simulink model "DTNS_SIM2"  (R2022a)
settings: Solver=ode4  StartTime=0.0  StopTime=100  FixedStep=0.01  RelTol=1e-3  EnableMultiTasking=on
PreLoadFcn:
  | listing = dir;
  | if (contains([listing.name], 'MAP')) &&  (contains([listing.name], 'DTNS_SIM.slx'))
  |     addpath('./AGR', './TRN', './TCAF', './FTG', './DYN', './FLCC', './GPS', './RALT', './INS', './MAP');
  |     addpath('./MAP/MAP_DB');
  | else
  |     warning('[DTNS_SIM.slx]는 DTNS 프로젝트 최상단 경로에 위치해야 합니다.');
  | end
  | 
  | load('BUS_STRUCTURE_DYN.mat');
  | load('BUS_STRUCTURE_FLCC.mat');
  | load('BUS_STRUCTURE_RALT.mat');
  | load('BUS_STRUCTURE_INS.mat');
  | load('BUS_STRUCTURE_GPS.mat');
  | load('BusStructureTRN.mat');
  | load('BusStructureLOSR.mat');
  | load('BusStructureHR.mat');
  | load('BusStructureCR.mat');
  | FTG_initState;
InitFcn:
  | listing = dir;
  | if (contains([listing.name], 'MAP')) &&  (contains([listing.name], 'DTNS_SIM.slx'))
  |     addpath('./AGR', './TRN', './TCAF', './FTG', './DYN', './FLCC', './GPS', './RALT', './INS', './MAP');
  |     addpath('./MAP/MAP_DB');
  | else
  |     warning('[DTNS_SIM.slx]는 DTNS 프로젝트 최상단 경로에 위치해야 합니다.');
  | end
  | 
  | load('BUS_STRUCTURE_DYN.mat');
  | load('BUS_STRUCTURE_FLCC.mat');
  | load('BUS_STRUCTURE_RALT.mat');
  | load('BUS_STRUCTURE_INS.mat');
  | load('BUS_STRUCTURE_GPS.mat');
  | load('BusStructureTRN.mat');
  | load('BusStructureLOSR.mat');
  | load('BusStructureHR.mat');
  | load('BusStructureCR.mat');
  | FTG_initState;
libraries: aerolibconvert2 x14, simulink_extras x5
(part 1 of 2)
settings Model: PacingRate=3  Creator=ASCL  LastModifiedBy=ASCL
settings SolverCC: PositivePriorityOrder=on  AutoInsertRateTranBlk=on
settings DataIOCC: ExternalInput=FTGScenario.getElement('IN_STICK'), [], [], FTGScenario.getElement('IN_FLIGHT_CMD'), []  LoadExternalInput=on  SaveOutput=off  DSMLogging=off  ReturnWorkspaceOutputs=off
settings OptimizationCC: BlockReduction=off  DefaultParameterBehavior=Inlined  UseDivisionForNetSlopeComputation=on  GainParamInheritBuiltInType=on  UseFloatMulNetSlope=on  ExpressionFolding=off  PassReuseOutputArgsAs=Individual arguments  ZeroExternalMemoryAtStartup=off  ZeroInternalMemoryAtStartup=off  EfficientFloat2IntCast=on  LifeSpan=inf  OptimizeBlockOrder=speed  DifferentSizesBufferReuse=on  EfficientTunableParamExpr=on
settings DebuggingCC: SignalInfNanChecking=warning  ReadBeforeWriteMsg=EnableAllAsError  WriteAfterWriteMsg=EnableAllAsError  WriteAfterReadMsg=EnableAllAsError  IntegerOverflowMsg=error  ParameterTunabilityLossMsg=error  UniqueDataStoreMsg=error  AssertControl=DisableAll  NonBusSignalsTreatedAsBus=error  SFInvalidInputDataAccessInChartInitDiag=error  SFTransitionOutsideNaturalParentDiag=error  SFUnreachableExecutionPathDiag=error  SFUndirectedBroadcastEventsDiag=error  IntegerSaturationMsg=error
settings HardwareCC: ProdBitPerPointer=32  ProdBitPerSizeT=32  ProdBitPerPtrDiffT=32  ProdLargestAtomicInteger=Long  ProdLargestAtomicFloat=Double  ProdEndianess=BigEndian  ProdWordSize=32  ProdLongLongMode=on  ProdHWDeviceType=Freescale->MPC83xx
settings ModelReferenceCC: ModelReferenceNumInstancesAllowed=Single
settings SFSimCC: SimCustomHeaderCode="#include \"MAP.h\""  SimUserSources=MAP.c  SimUserLibraries=WS2_32.LIB  CompileTimeRecursionLimit=0  EnableRuntimeRecursion=off  MATLABDynamicMemAlloc=off  CustomCodeGlobalsAsFunctionIO=on
settings RTWCC: SystemTargetFile=ert.tlc  TemplateMakefile=ert_default_tmf  GenerateReport=on  RTWUseSimCustomCode=on  CustomHeaderCode="#include \"MAP.h\""  CustomSource=MAP.c  CustomLibrary=WS2_32.LIB  BuildConfiguration=Faster Runs  IncludeHyperlinkInReport=on  LaunchReport=on  GenerateTraceInfo=on  GenerateTraceReport=on  GenerateTraceReportSl=on  GenerateTraceReportSf=on  GenerateTraceReportEml=on  GenerateCodeMetricsReport=on
settings CodeAppCC: ForceParamTrailComments=on  IgnoreCustomStorageClasses=off  OperatorAnnotations=on  SimulinkDataObjDesc=on  SFDataObjDesc=on  MATLABFcnDesc=on  InsertBlockDesc=on  StateflowObjectComments=on  MATLABSourceComments=on  EnableCustomComments=on  InlinedPrmAccess=Macros  ReqsInCode=on
settings ERTTargetCC: TargetLangStandard=C99 (ISO)  UtilityFuncGeneration=Shared location  GenerateSampleERTMain=on  CombineSignalStateStructs=on  SuppressErrorStatus=on  SupportNonFinite=off  SupportVariableSizeSignals=on  ParenthesesLevel=Standards  CastingMode=Standards  GenerateSharedConstants=off  InlinedParameterPlacement=NonHierarchical  ERTCustomFileTemplate=example_file_process.tlc  RateTransitionBlockCode=Function  PreserveIfCondition=on  ConvertIfToSwitch=off  EnableSignedLeftShifts=off  EnableSignedRightShifts=off

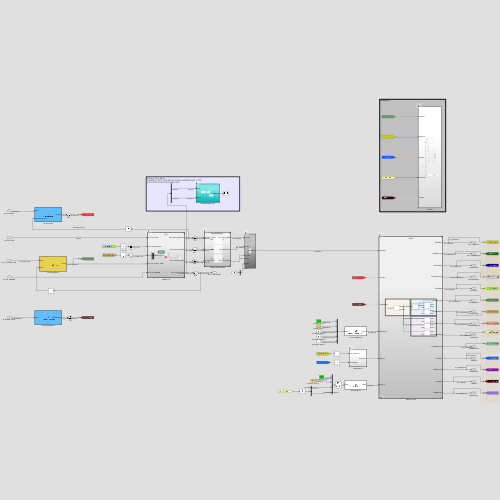
[thumbnail: Simulink's stored preview of the top-level diagram]
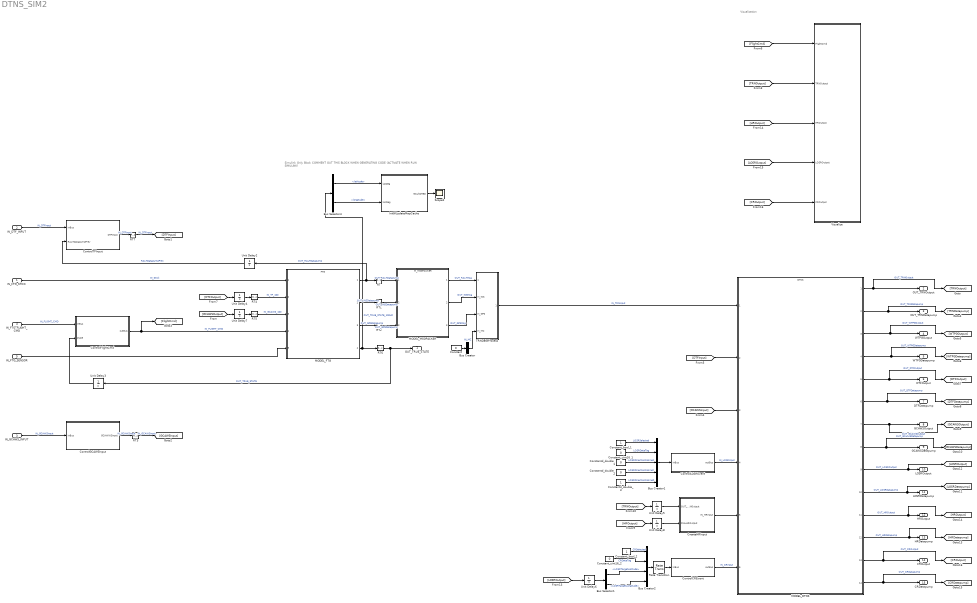
== system DTNS_SIM2 ==
  note: Visualization
  note: Simulink Only Block
      | COMMENT OUT THIS BLOCK WHEN GENERATING CODE
      | (ACTIVATE WHEN RUN SIMULINK)
  IN_FTG_STICK : Inport  OutDataTypeStr=Bus: BUS_FLCC_STICK  BusOutputAsStruct=on
  IN_DTF_INPUT : Inport  Port=2  OutDataTypeStr=Bus: DTFInput  BusOutputAsStruct=on
  IN_GCAWS_INPUT : Inport  Port=3  OutDataTypeStr=Bus: GCAWSInput  BusOutputAsStruct=on
  IN_FTG_FLIGHT_CMD : Inport  Port=4  OutDataTypeStr=Bus: BUS_FLCC_FLIGHT_CMD  Interpolate=off  BusOutputAsStruct=on
  IN_FTG_SENSOR : Inport  Port=5  OutDataTypeStr=Bus: BUS_SENSOR_ALL_INPUTSTATUS  BusOutputAsStruct=on
  Bus Creator : BusCreator  Inputs=1  OutDataTypeStr=Bus: TRN_MC  NonVirtualBus=on
      settings: InheritFromInputs=off
  Bus Creator1 : BusCreator  Inputs=5  OutDataTypeStr=Bus: LOSRInput  NonVirtualBus=on
      settings: InheritFromInputs=off
  Bus Creator2 : BusCreator  Inputs=4  OutDataTypeStr=Bus: CRInput
      settings: InheritFromInputs=off
  Bus Selector1 : BusSelector  OutputSignals=LOSRTargetLatitude,LOSRTargetLongitude
  Bus Selector4 : BusSelector  OutputSignals=latitude,longitude
  Constant : Constant  Value=0  OutDataTypeStr=boolean  SampleTime=0.04
  Constant_bool_1 : Constant  OutDataTypeStr=boolean  SampleTime=0.04
  Constant_bool_2 : Constant  OutDataTypeStr=boolean  SampleTime=0.04
  Constant_uint16_1 : Constant  Value=0  OutDataTypeStr=uint16  SampleTime=0.04
  Constant_uint16_2 : Constant  Value=0  OutDataTypeStr=uint16  SampleTime=0.04
  Constantd_double_1 : Constant  Value=0  OutDataTypeStr=double  SampleTime=0.04
  Constantd_double_2 : Constant  Value=0  OutDataTypeStr=double  SampleTime=0.04
  Constantd_double_3 : Constant  OutDataTypeStr=double  SampleTime=0.04
  ControlCREvent : MATLAB Function  TreatAsAtomicUnit=on  SystemSampleTime=0.04
  ControlFlightCmd : MATLAB Function  TreatAsAtomicUnit=on  SystemSampleTime=0.01
  ControlGCAWSInput : MATLAB Function  TreatAsAtomicUnit=on  SystemSampleTime=0.01
  ControlLOSREvent : MATLAB Function  TreatAsAtomicUnit=on  SystemSampleTime=0.04
  ControlTFInput : MATLAB Function  TreatAsAtomicUnit=on  SystemSampleTime=0.01
  CreateHRInput : Subsystem  TreatAsAtomicUnit=on  ScheduleAs=Periodic partition  PartitionName=CreateHRInput  SystemSampleTime=0.04
      settings: RTWSystemCode=Nonreusable function
  InitNUpdateMapCache : Subsystem  TreatAsAtomicUnit=on  ScheduleAs=Periodic partition  PartitionName=InitNUpdateMapCache  SystemSampleTime=0.01
  MODEL_DTNS : ModelReference  ModelNameDialog=DTNS.slx  SimulationMode=Normal  ScheduleRates=on  ScheduleRatesWith=Schedule Editor  ModelReferenceVersion=1.240
  MODEL_FTG : ModelReference  ModelNameDialog=FTG.slx  SimulationMode=Normal  ScheduleRates=on  ScheduleRatesWith=Schedule Editor  ModelReferenceVersion=1.515
  MODEL_MSGPACKER : ModelReference  ModelNameDialog=M_MSGPACKER.slx  SimulationMode=Normal  ScheduleRates=on  ScheduleRatesWith=Schedule Editor  ModelReferenceVersion=1.319
  RT{,1..3,6..7} (6 alike) : RateTransition  OutPortSampleTime=0.04
  RT4 : RateTransition  OutPortSampleTime=0.01
  RT5 : RateTransition  OutPortSampleTime=0.01
  Rate Transition : RateTransition  OutPortSampleTime=0.04
  Scope2 : Scope
  TRNDataProcess : Subsystem  TreatAsAtomicUnit=on  ScheduleAs=Periodic partition  PartitionName=TRNDataProcess  SystemSampleTime=0.04
  Unit Delay2 : UnitDelay  SampleTime=0.01  HasFrameUpgradeWarning=on
  Unit Delay3 : UnitDelay  SampleTime=-1  HasFrameUpgradeWarning=on
  Unit Delay{4..8} (5 alike) : UnitDelay  SampleTime=0.04  HasFrameUpgradeWarning=on
  Visualize : Subsystem  TreatAsAtomicUnit=on  ScheduleAs=Periodic partition  PartitionName=Visualize  SystemSampleTime=0.04
  OUT_TRUE_STATE : Outport  OutDataTypeStr=Bus: BUS_DYN_STATE  BusOutputAsStruct=on
  OUT_TRNOutput : Outport  Port=2  OutDataTypeStr=Bus: TRNOutput  SampleTime=0.04
  OUT_TRNDatapump : Outport  Port=3  OutDataTypeStr=Bus: TRNDatapump  SampleTime=0.04
  WTPGOutput : Outport  Port=4  OutDataTypeStr=Bus: WTPGOutput  SampleTime=0.04
  WTPGDatapump : Outport  Port=5  OutDataTypeStr=Bus: WTPGDatapump  SampleTime=0.04
  DTFOutput : Outport  Port=6  OutDataTypeStr=Bus: DTFOutput  SampleTime=0.04
  DTFDatapump : Outport  Port=7  OutDataTypeStr=Bus: DTFDatapump  SampleTime=0.04
  GCAWSOutput : Outport  Port=8  OutDataTypeStr=Bus: GCAWSOutput  SampleTime=0.04
  GCAWSDatapump : Outport  Port=9  OutDataTypeStr=Bus: GCAWSDatapump  SampleTime=0.04
  LOSROutput : Outport  Port=10  OutDataTypeStr=Bus: LOSROutput  SampleTime=0.04  BusOutputAsStruct=on
  LOSRDatapump : Outport  Port=11  OutDataTypeStr=Bus: LOSRDatapump  SampleTime=0.04  BusOutputAsStruct=on
  HROutput : Outport  Port=12  OutDataTypeStr=Bus: HROutput  SampleTime=0.04  BusOutputAsStruct=on
  HRDatapump : Outport  Port=13  OutDataTypeStr=Bus: HRDatapump  SampleTime=0.04  BusOutputAsStruct=on
  CROutput : Outport  Port=14  OutDataTypeStr=Bus: CROutput  SampleTime=0.04  BusOutputAsStruct=on
  CRDatapump : Outport  Port=15  OutDataTypeStr=Bus: CRDatapump  SampleTime=0.04  BusOutputAsStruct=on
  wires:
  Bus Creator/1 -> TRNDataProcess/4(In_MC)  "IN_MC"
  MODEL_FTG/3 -> RT2/1  "OUT_GPSDatapump"
  MODEL_DTNS/4 -> [WTPGDatapump], WTPGDatapump/1  "OUT_WTPGDatapump"
  MODEL_DTNS/8 -> [GCAWSDatapump], GCAWSDatapump/1  "OUT_GCAWSDatapump"
  MODEL_DTNS/2 -> [TRNDatapump], OUT_TRNDatapump/1  "OUT_TRNDatapump"
  MODEL_DTNS/7 -> GCAWSOutput/1, [GCAWSOutput]  "OUT_GCAWSOutput"
  Constant/1 -> Bus Creator/1
  IN_GCAWS_INPUT/1 -> ControlGCAWSInput/1(inBus)  "IN_GCAWSInput"
  IN_FTG_FLIGHT_CMD/1 -> ControlFlightCmd/1(inBus)  "IN_FLIGHT_CMD"
  RT6/1 -> Unit Delay3/1, OUT_TRUE_STATE/1  "OUT_TRUE_STATE"
  Bus Selector4/2 -> InitNUpdateMapCache/2(lonDeg)  "<longitude>"
  MODEL_FTG/2 -> RT1/1  "OUT_INSDatapump"
  MODEL_FTG/1 -> RT/1, Unit Delay2/1  "OUT_RALTDatapump"
  IN_FTG_STICK/1 -> MODEL_FTG/1  "IN_Stick"
  MODEL_DTNS/5 -> DTFOutput/1, [DTFOutput]  "OUT_DTFOutput"
  ControlFlightCmd/1(outBus) -> MODEL_FTG/4, [FlightCmd]  "IN_FLIGHT_CMD"
  IN_DTF_INPUT/1 -> ControlTFInput/1(inBus)  "IN_DTFInput"
  MODEL_MSGPACKER/3 -> TRNDataProcess/3(In_GPS)  "OUT_GPSMsg"
  MODEL_MSGPACKER/1 -> TRNDataProcess/1(In_RALT)  "OUT_RALTMsg"
  MODEL_MSGPACKER/2 -> TRNDataProcess/2(In_INS)  "OUT_INSMsg"
  InitNUpdateMapCache/1(resultDTED) -> Scope2/1
  IN_FTG_SENSOR/1 -> MODEL_FTG/5
  RT7/1 -> [DTFInput]  "IN_DTFInput"
  Unit Delay2/1 -> ControlTFInput/2(RALTDatapumpPrev)  "RALTDatapumpPrev"
  RT3/1 -> [GCAWSInput]  "IN_GCAWSInput"
  Unit Delay3/1 -> ControlFlightCmd/2(state)
  TRNDataProcess/1(TRN INPUT) -> MODEL_DTNS/1  "IN_TRNInput"
  RT/1 -> MODEL_MSGPACKER/1  "OUT_RALTDatapump"
  RT1/1 -> MODEL_MSGPACKER/2  "OUT_INSDatapump"
  RT2/1 -> MODEL_MSGPACKER/3  "OUT_GPSDatapump"
  Bus Selector4/1 -> InitNUpdateMapCache/1(latDeg)  "<latitude>"
  RT4/1 -> MODEL_FTG/2  "IN_TF_100"
  RT5/1 -> MODEL_FTG/3  "IN_GCAWS_100"
  MODEL_FTG/4 -> Bus Selector4/1, RT6/1  "OUT_TRUE_STATE_100HZ"
  MODEL_DTNS/12 -> [HRDatapump], HRDatapump/1  "OUT_HRDatapump"
  Bus Creator1/1 -> ControlLOSREvent/1(inBus)
  Constant_uint16_1/1 -> Bus Creator1/2  "LOSRDataTag"
  MODEL_DTNS/9 -> LOSROutput/1, [LOSROutput]  "OUT_LOSROutput"
  MODEL_DTNS/1 -> [TRNOutput], OUT_TRNOutput/1  "OUT_TRNOutput"
  MODEL_DTNS/14 -> [CRDatapump], CRDatapump/1  "OUT_CRDatapump"
  MODEL_DTNS/13 -> [CROutput], CROutput/1  "OUT_CROutput"
  Constantd_double_2/1 -> Bus Creator1/4  "LOSRDirectionCosineY"
  Constant_bool_1/1 -> Bus Creator1/1  "LOSRSelected"
  ControlLOSREvent/1(outBus) -> MODEL_DTNS/4  "IN_LOSRInput"
  Constantd_double_3/1 -> Bus Creator1/5  "LOSRDirectionCosineZ"
  Constantd_double_1/1 -> Bus Creator1/3  "LOSRDirectionCosineX"
  MODEL_DTNS/10 -> [LOSRDatapump], LOSRDatapump/1  "OUT_LOSRDatapump"
  MODEL_DTNS/6 -> [DTFDatapump], DTFDatapump/1  "OUT_DTFDatapump"
  CreateHRInput/1(IN_HRInput) -> MODEL_DTNS/5
  MODEL_DTNS/3 -> [WTPGOutput], WTPGOutput/1  "OUT_WTPGOutput"
  MODEL_DTNS/11 -> [HROutput], HROutput/1  "OUT_HROutput"
  [TRNOutput] -> Visualize/2(TRNOutput)
  [FlightCmd] -> Visualize/1(FlightCmd)
  [HROutput] -> Visualize/3(HROutput)
  [LOSROutput] -> Visualize/4(LOSROutput)
  [CROutput] -> Visualize/5(CROutput)
  [TRNOutput] -> Unit Delay5/1
  ControlGCAWSInput/1(GCAWWSInput) -> RT3/1  "IN_GCAWSInput"
  ControlTFInput/1(DTFInput) -> RT7/1  "IN_DTFInput"
  [DTFInput] -> MODEL_DTNS/2
  [GCAWSInput] -> MODEL_DTNS/3
  Unit Delay5/1 -> CreateHRInput/1(OUT_TRNOutput)
  Bus Selector1/2 -> Bus Creator2/4  "<LOSRTargetLongitude>"
  [LOSROutput] -> Unit Delay6/1
  Rate Transition/1 -> ControlCREvent/1(inBus)
  Bus Selector1/1 -> Bus Creator2/3  "<LOSRTargetLatitude>"
  Bus Creator2/1 -> Rate Transition/1
  ControlCREvent/1(outBus) -> MODEL_DTNS/6  "IN_CRInput"
  Constant_bool_2/1 -> Bus Creator2/1  "CRSelected"
  Constant_uint16_2/1 -> Bus Creator2/2  "CRDataTag"
  Unit Delay6/1 -> Bus Selector1/1
  [DTFOutput] -> Unit Delay4/1
  Unit Delay4/1 -> RT4/1
  Unit Delay7/1 -> RT5/1
  [HROutput] -> Unit Delay8/1
  Unit Delay8/1 -> CreateHRInput/2(PrevHROutput)
  [GCAWSOutput] -> Unit Delay7/1

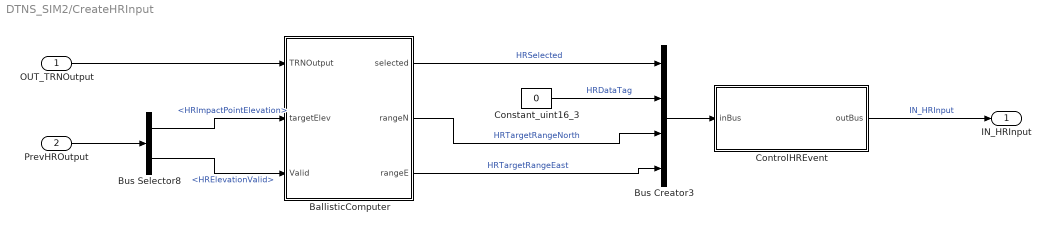
== system DTNS_SIM2/CreateHRInput ==
  OUT_TRNOutput : Inport
  PrevHROutput : Inport  Port=2
  BallisticComputer : MATLAB Function  TreatAsAtomicUnit=on  SystemSampleTime=0.04
  Bus Creator3 : BusCreator  Inputs=4  OutDataTypeStr=Bus: HRInput  NonVirtualBus=on
      settings: InheritFromInputs=off
  Bus Selector8 : BusSelector  OutputSignals=HRImpactPointElevation,HRElevationValid
  Constant_uint16_3 : Constant  Value=0  OutDataTypeStr=uint16  SampleTime=0.04
  ControlHREvent : MATLAB Function  TreatAsAtomicUnit=on  SystemSampleTime=0.04
  IN_HRInput : Outport
  wires:
  BallisticComputer/3(rangeE) -> Bus Creator3/4  "HRTargetRangeEast"
  BallisticComputer/2(rangeN) -> Bus Creator3/3  "HRTargetRangeNorth"
  Bus Selector8/1 -> BallisticComputer/2(targetElev)  "<HRImpactPointElevation>"
  BallisticComputer/1(selected) -> Bus Creator3/1  "HRSelected"
  OUT_TRNOutput/1 -> BallisticComputer/1(TRNOutput)
  Constant_uint16_3/1 -> Bus Creator3/2  "HRDataTag"
  Bus Creator3/1 -> ControlHREvent/1(inBus)
  Bus Selector8/2 -> BallisticComputer/3(Valid)  "<HRElevationValid>"
  PrevHROutput/1 -> Bus Selector8/1
  ControlHREvent/1(outBus) -> IN_HRInput/1  "IN_HRInput"

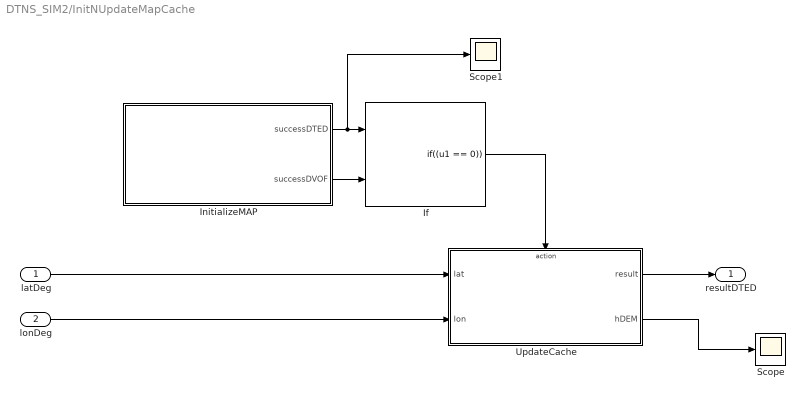
== system DTNS_SIM2/InitNUpdateMapCache ==
  latDeg : Inport  OutDataTypeStr=double
  lonDeg : Inport  Port=2  OutDataTypeStr=double
  If : If  NumInputs=2  IfExpression=(u1 == 0)  ShowElse=off
  InitializeMAP : MATLAB Function  TreatAsAtomicUnit=on
  Scope : Scope
  Scope1 : Scope
  UpdateCache : Subsystem  TreatAsAtomicUnit=on
  resultDTED : Outport  VectorParamsAs1DForOutWhenUnconnected=off
  wires:
  lonDeg/1 -> UpdateCache/2(lon)
  UpdateCache/1(result) -> resultDTED/1
  InitializeMAP/1(successDTED) -> Scope1/1, If/1
  latDeg/1 -> UpdateCache/1(lat)
  InitializeMAP/2(successDVOF) -> If/2
  If/1 -> UpdateCache/Action
  UpdateCache/2(hDEM) -> Scope/1

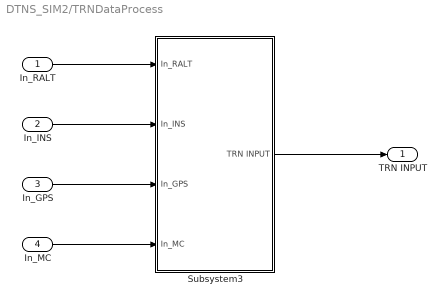
== system DTNS_SIM2/TRNDataProcess ==
  In_RALT : Inport  SampleTime=0.04
  In_INS : Inport  Port=2  SampleTime=0.04
  In_GPS : Inport  Port=3  SampleTime=0.04
  In_MC : Inport  Port=4  SampleTime=0.04
  Subsystem3 : Subsystem
  TRN INPUT : Outport  SampleTime=0.04
  wires:
  In_GPS/1 -> Subsystem3/3(In_GPS)
  In_MC/1 -> Subsystem3/4(In_MC)
  Subsystem3/1(TRN INPUT) -> TRN INPUT/1
  In_RALT/1 -> Subsystem3/1(In_RALT)
  In_INS/1 -> Subsystem3/2(In_INS)

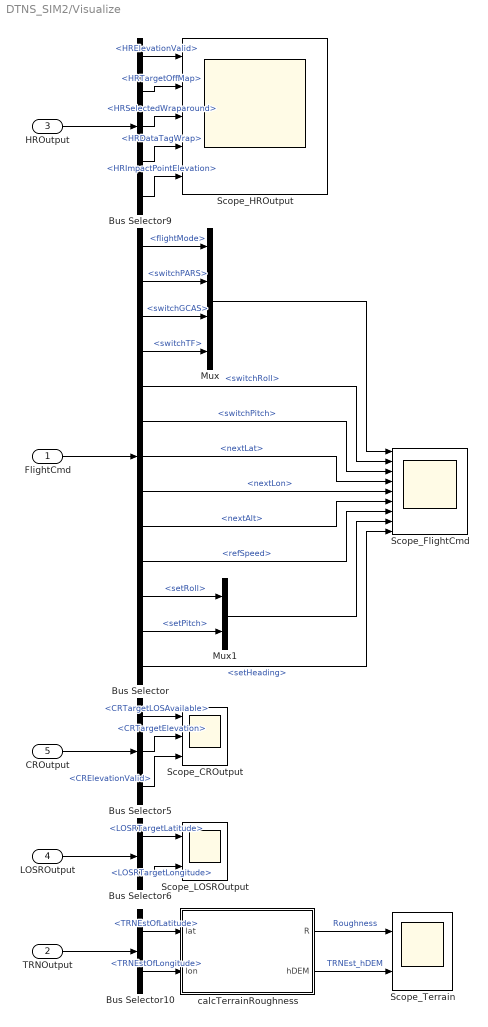
== system DTNS_SIM2/Visualize ==
  FlightCmd : Inport
  TRNOutput : Inport  Port=2
  HROutput : Inport  Port=3
  LOSROutput : Inport  Port=4
  CROutput : Inport  Port=5
  Bus Selector : BusSelector  OutputSignals=flightMode,switchPARS,switchGCAS,switchTF,switchRoll,switchPitch,nextLat,nextLon,nextAlt,refSpeed,setRoll,setPitch,setHeading
  Bus Selector10 : BusSelector  OutputSignals=TRNEstOfLatitude,TRNEstOfLongitude
  Bus Selector5 : BusSelector  OutputSignals=CRTargetLOSAvailable,CRTargetElevation,CRElevationValid
  Bus Selector6 : BusSelector  OutputSignals=LOSRTargetLatitude,LOSRTargetLongitude
  Bus Selector9 : BusSelector  OutputSignals=HRElevationValid,HRTargetOffMap,HRSelectedWraparound,HRDataTagWrap,HRImpactPointElevation
  Mux : Mux
  Mux1 : Mux  Inputs=2
  Scope_CROutput : Scope  NumInputPorts=3
  Scope_FlightCmd : Scope  NumInputPorts=9
  Scope_HROutput : Scope  NumInputPorts=5
  Scope_LOSROutput : Scope  NumInputPorts=2
  Scope_Terrain : Scope  NumInputPorts=2
  calcTerrainRoughness : MATLAB Function  TreatAsAtomicUnit=on
  wires:
  calcTerrainRoughness/2(hDEM) -> Scope_Terrain/2  "TRNEst_hDEM"
  FlightCmd/1 -> Bus Selector/1
  HROutput/1 -> Bus Selector9/1
  Bus Selector5/1 -> Scope_CROutput/1  "<CRTargetLOSAvailable>"
  Bus Selector9/5 -> Scope_HROutput/5  "<HRImpactPointElevation>"
  Bus Selector9/3 -> Scope_HROutput/3  "<HRSelectedWraparound>"
  Bus Selector10/1 -> calcTerrainRoughness/1(lat)  "<TRNEstOfLatitude>"
  Bus Selector6/2 -> Scope_LOSROutput/2  "<LOSRTargetLongitude>"
  Bus Selector10/2 -> calcTerrainRoughness/2(lon)  "<TRNEstOfLongitude>"
  Bus Selector5/3 -> Scope_CROutput/3  "<CRElevationValid>"
  Bus Selector5/2 -> Scope_CROutput/2  "<CRTargetElevation>"
  Bus Selector9/1 -> Scope_HROutput/1  "<HRElevationValid>"
  Bus Selector/6 -> Scope_FlightCmd/3  "<switchPitch>"
  Bus Selector/10 -> Scope_FlightCmd/7  "<refSpeed>"
  Bus Selector9/4 -> Scope_HROutput/4  "<HRDataTagWrap>"
  Bus Selector/7 -> Scope_FlightCmd/4  "<nextLat>"
  TRNOutput/1 -> Bus Selector10/1
  Bus Selector6/1 -> Scope_LOSROutput/1  "<LOSRTargetLatitude>"
  Bus Selector/11 -> Mux1/1  "<setRoll>"
  Mux/1 -> Scope_FlightCmd/1
  Bus Selector/12 -> Mux1/2  "<setPitch>"
  Bus Selector/8 -> Scope_FlightCmd/5  "<nextLon>"
  Bus Selector/4 -> Mux/4  "<switchTF>"
  Bus Selector/13 -> Scope_FlightCmd/9  "<setHeading>"
  Bus Selector/9 -> Scope_FlightCmd/6  "<nextAlt>"
  Bus Selector/5 -> Scope_FlightCmd/2  "<switchRoll>"
  Bus Selector9/2 -> Scope_HROutput/2  "<HRTargetOffMap>"
  Bus Selector/1 -> Mux/1  "<flightMode>"
  CROutput/1 -> Bus Selector5/1
  Bus Selector/2 -> Mux/2  "<switchPARS>"
  Mux1/1 -> Scope_FlightCmd/8
  Bus Selector/3 -> Mux/3  "<switchGCAS>"
  LOSROutput/1 -> Bus Selector6/1
  calcTerrainRoughness/1(R) -> Scope_Terrain/1  "Roughness"

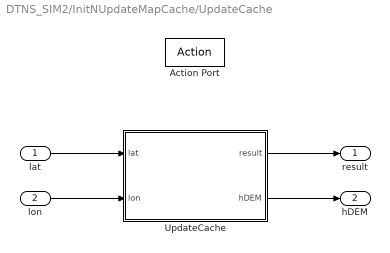
== system DTNS_SIM2/InitNUpdateMapCache/UpdateCache ==
  lat : Inport
  lon : Inport  Port=2
  Action Port : ActionPort  ActionPortLabel=if((u1 == 0))
  UpdateCache : MATLAB Function  TreatAsAtomicUnit=on
  result : Outport  VectorParamsAs1DForOutWhenUnconnected=off
  hDEM : Outport  Port=2
  wires:
  UpdateCache/1(result) -> result/1
  lat/1 -> UpdateCache/1(lat)
  lon/1 -> UpdateCache/2(lon)
  UpdateCache/2(hDEM) -> hDEM/1

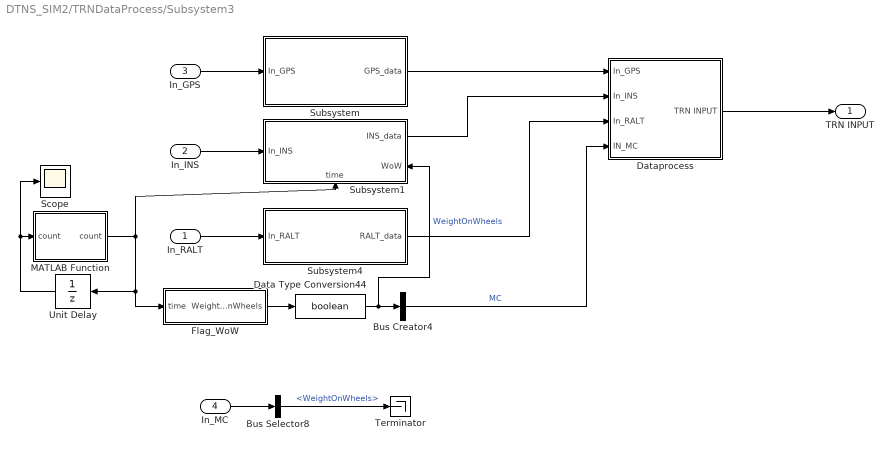
== system DTNS_SIM2/TRNDataProcess/Subsystem3 ==
  In_RALT : Inport  SampleTime=0.04
  In_INS : Inport  Port=2  SampleTime=0.04
  In_GPS : Inport  Port=3  SampleTime=0.04
  In_MC : Inport  Port=4  SampleTime=0.04
  Bus Creator4 : BusCreator  Inputs=1  OutDataTypeStr=Bus: TRN_MC  NonVirtualBus=on
      settings: InheritFromInputs=off
  Bus Selector8 : BusSelector  OutputSignals=WeightOnWheels
  Data Type Conversion44 : DataTypeConversion  OutDataTypeStr=boolean  SaturateOnIntegerOverflow=off  RndMeth=Floor
  Dataprocess : Subsystem
  Flag_WoW : MATLAB Function  TreatAsAtomicUnit=on  SystemSampleTime=0.04
  MATLAB Function : MATLAB Function  TreatAsAtomicUnit=on  SystemSampleTime=0.04
  Scope : Scope
  Subsystem : Subsystem
  Subsystem1 : Subsystem
      settings: PortSchema="{\"entries\":[{\"content\":{\"sides\":[{\"content\":{\"connectorIds\":[\"In1\"]},\"type\":\"ConnectorPlacement.EquallySpacedRectSide\",\"uuid\":\"627687e9-0c69-45fe-ab30-f2b8c78c94c9\"},{\"content\":{\"connectorIds\":[\"Out1\",\"In3\"],\"side\":\"RIGHT\"},\"type\":\"ConnectorPlacement.EquallySpacedRectSide\",\"uuid\":\"cca5eff4-b683-4134-86dd-9b38fc1aef42\"},{\"content\":{\"connectorIds\":[],\"side\":\"TOP\"},\"type\":\"ConnectorPlacement.EquallySpacedRectSide\",\"uuid\":\"db09404b-1405-40a7-9047-09d57f6d1ee9\"},{\"content\":{\"connectorIds\":[\"In2\"],\"side\":\"BOTTOM\"},\"type\":\"ConnectorPlacement.EquallySpacedRectSide\",\"uuid\":\"43181e0c-7a64-4398-bddd-a3419aca840e\"}]},\"type\":\"ConnectorPlacement.EquallySpacedConnector\",\"uuid\":\"8e5a566a-2f6b-4dcc-950b-8518900682ca\"}],\"packageUris\":[\"http://schema.mathworks.com/mf0/Connector/R2020b\"],\"version\":\"1.0\"}"
  Subsystem4 : Subsystem
  Terminator : Terminator
  Unit Delay : UnitDelay  SampleTime=0.04  HasFrameUpgradeWarning=on
  TRN INPUT : Outport  SampleTime=0.04
  wires:
  Flag_WoW/1(WeightOnWheels) -> Data Type Conversion44/1
  Data Type Conversion44/1 -> Subsystem1/3(WoW), Bus Creator4/1  "WeightOnWheels"
  Subsystem1/1(INS_data) -> Dataprocess/2(In_INS)
  Bus Creator4/1 -> Dataprocess/4(IN_MC)  "MC"
  Subsystem/1(GPS_data) -> Dataprocess/1(In_GPS)
  Dataprocess/1(TRN INPUT) -> TRN INPUT/1
  In_MC/1 -> Bus Selector8/1
  In_GPS/1 -> Subsystem/1(In_GPS)
  In_INS/1 -> Subsystem1/1(In_INS)
  In_RALT/1 -> Subsystem4/1(In_RALT)
  Subsystem4/1(RALT_data) -> Dataprocess/3(In_RALT)
  MATLAB Function/1(count) -> Unit Delay/1, Flag_WoW/1(time), Subsystem1/2(time)
  Unit Delay/1 -> Scope/1, MATLAB Function/1("count ")
  Bus Selector8/1 -> Terminator/1  "<WeightOnWheels>"

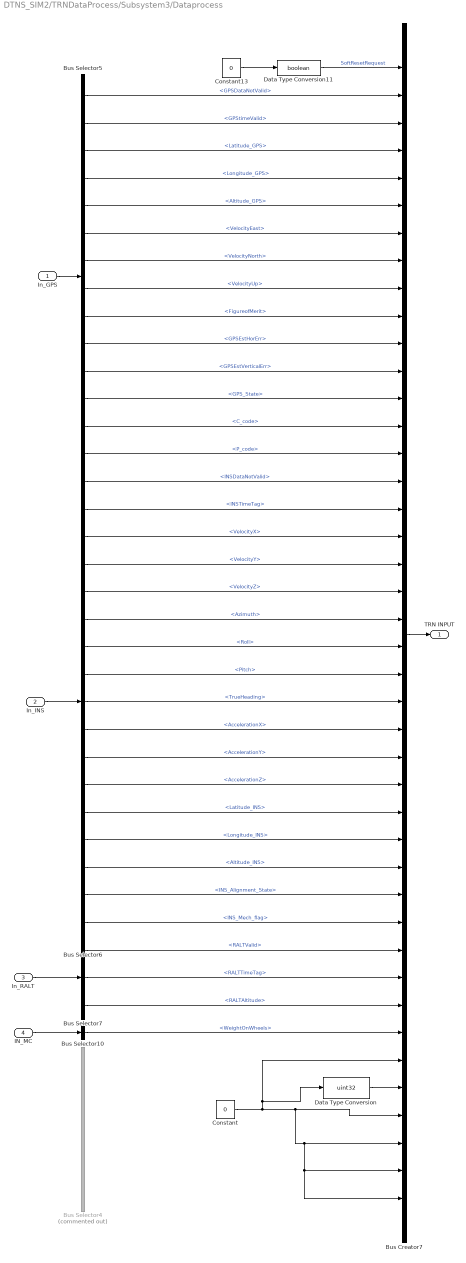
== system DTNS_SIM2/TRNDataProcess/Subsystem3/Dataprocess ==
  In_GPS : Inport  SampleTime=0.04
  In_INS : Inport  Port=2  SampleTime=0.04
  In_RALT : Inport  Port=3  SampleTime=0.04
  IN_MC : Inport  Port=4  SampleTime=0.04
  Bus Creator7 : BusCreator  Inputs=42  OutDataTypeStr=Bus: TRNInput  NonVirtualBus=on
      settings: InheritFromInputs=off
  Bus Selector10 : BusSelector  OutputSignals=WeightOnWheels
  Bus Selector4 : BusSelector  Commented=on  OutputSignals=MAP_hight,Map_Level,Map_size,Map_resolution,bottomLat,leftLon
  Bus Selector5 : BusSelector  OutputSignals=GPSDataNotValid,GPStimeValid,Latitude_GPS,Longitude_GPS,Altitude_GPS,VelocityEast,VelocityNorth,VelocityUp,FigureofMerit,GPSEstHorErr,GPSEstVerticalErr,GPS_State,C_code,P_code
  Bus Selector6 : BusSelector  OutputSignals=INSDataNotValid,INSTimeTag,VelocityX,VelocityY,VelocityZ,Azimuth,Roll,Pitch,TrueHeading,AccelerationX,AccelerationY,AccelerationZ,Latitude_INS,Longitude_INS,Altitude_INS,INS_Alignment_State,INS_Mech_flag
  Bus Selector7 : BusSelector  OutputSignals=RALTValid,RALTTimeTag,RALTAltitude
  Constant : Constant  Value=0  SampleTime=0.04
  Constant13 : Constant  Value=0  SampleTime=0.04
  Data Type Conversion : DataTypeConversion  OutDataTypeStr=uint32  SaturateOnIntegerOverflow=off  RndMeth=Floor
  Data Type Conversion11 : DataTypeConversion  OutDataTypeStr=boolean  SaturateOnIntegerOverflow=off  RndMeth=Floor
  TRN INPUT : Outport  OutDataTypeStr=Bus: TRNInput  SampleTime=0.04  VectorParamsAs1DForOutWhenUnconnected=off
  wires:
  Bus Selector5/8 -> Bus Creator7/9  "<VelocityUp>"
  Bus Selector6/16 -> Bus Creator7/31  "<INS_Alignment_State>"
  Bus Selector5/7 -> Bus Creator7/8  "<VelocityNorth>"
  In_GPS/1 -> Bus Selector5/1
  Bus Selector5/4 -> Bus Creator7/5  "<Longitude_GPS>"
  Bus Selector5/11 -> Bus Creator7/12  "<GPSEstVerticalErr>"
  Bus Selector5/3 -> Bus Creator7/4  "<Latitude_GPS>"
  Bus Selector6/13 -> Bus Creator7/28  "<Latitude_INS>"
  Bus Selector6/14 -> Bus Creator7/29  "<Longitude_INS>"
  Bus Selector5/12 -> Bus Creator7/13  "<GPS_State>"
  Bus Selector6/9 -> Bus Creator7/24  "<TrueHeading>"
  Bus Selector5/14 -> Bus Creator7/15  "<P_code>"
  Bus Selector6/1 -> Bus Creator7/16  "<INSDataNotValid>"
  Bus Creator7/1 -> TRN INPUT/1
  Data Type Conversion11/1 -> Bus Creator7/1  "SoftResetRequest"
  Bus Selector5/6 -> Bus Creator7/7  "<VelocityEast>"
  Bus Selector6/12 -> Bus Creator7/27  "<AccelerationZ>"
  Bus Selector6/3 -> Bus Creator7/18  "<VelocityX>"
  Bus Selector5/13 -> Bus Creator7/14  "<C_code>"
  Bus Selector6/6 -> Bus Creator7/21  "<Azimuth>"
  Bus Selector5/5 -> Bus Creator7/6  "<Altitude_GPS>"
  Bus Selector6/10 -> Bus Creator7/25  "<AccelerationX>"
  Bus Selector7/3 -> Bus Creator7/35  "<RALTAltitude>"
  In_INS/1 -> Bus Selector6/1
  Bus Selector7/1 -> Bus Creator7/33  "<RALTValid>"
  Bus Selector5/1 -> Bus Creator7/2  "<GPSDataNotValid>"
  Bus Selector10/1 -> Bus Creator7/36  "<WeightOnWheels>"
  Bus Selector6/17 -> Bus Creator7/32  "<INS_Mech_flag>"
  Bus Selector6/4 -> Bus Creator7/19  "<VelocityY>"
  Bus Selector6/7 -> Bus Creator7/22  "<Roll>"
  Constant13/1 -> Data Type Conversion11/1
  Bus Selector7/2 -> Bus Creator7/34  "<RALTTimeTag>"
  Bus Selector6/5 -> Bus Creator7/20  "<VelocityZ>"
  Bus Selector6/2 -> Bus Creator7/17  "<INSTimeTag>"
  Bus Selector6/8 -> Bus Creator7/23  "<Pitch>"
  Bus Selector5/2 -> Bus Creator7/3  "<GPStimeValid>"
  Bus Selector5/10 -> Bus Creator7/11  "<GPSEstHorErr>"
  Bus Selector6/15 -> Bus Creator7/30  "<Altitude_INS>"
  Bus Selector6/11 -> Bus Creator7/26  "<AccelerationY>"
  Bus Selector5/9 -> Bus Creator7/10  "<FigureofMerit>"
  In_RALT/1 -> Bus Selector7/1
  IN_MC/1 -> Bus Selector10/1
  Constant/1 -> Bus Creator7/39, Bus Creator7/40, Bus Creator7/42, Bus Creator7/41, Bus Creator7/37, Data Type Conversion/1
  Data Type Conversion/1 -> Bus Creator7/38

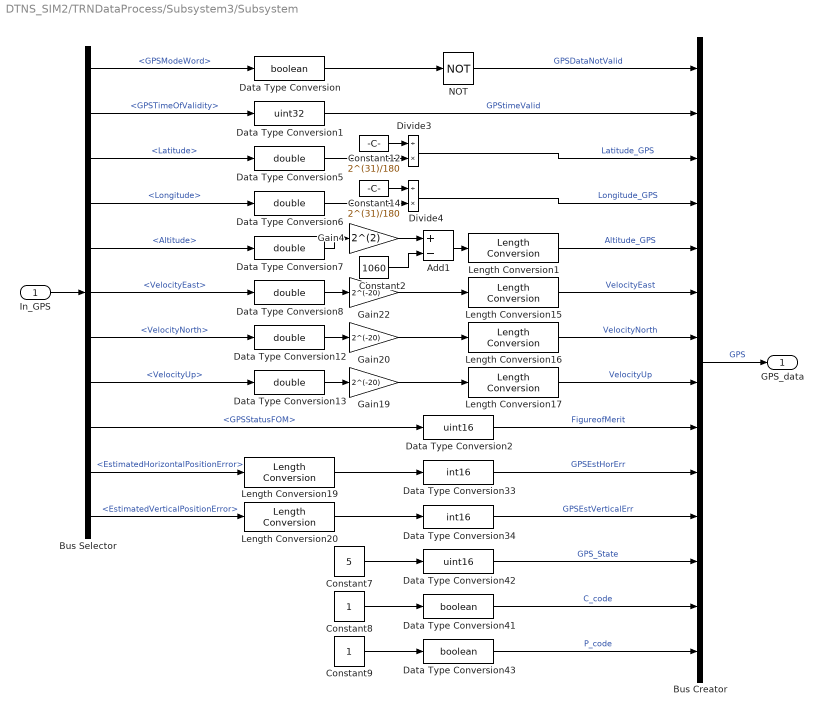
== system DTNS_SIM2/TRNDataProcess/Subsystem3/Subsystem ==
  In_GPS : Inport  SampleTime=0.04
  Add1 : Sum  Inputs=+-
  Bus Creator : BusCreator  Inputs=14  OutDataTypeStr=Bus: TRN_GPS  NonVirtualBus=on
      settings: InheritFromInputs=off
  Bus Selector : BusSelector  OutputSignals=GPSModeWord,GPSTimeOfValidity,Latitude,Longitude,Altitude,VelocityEast,VelocityNorth,VelocityUp,GPSStatusFOM,EstimatedHorizontalPositionError,EstimatedVerticalPositionError
  Constant12 : Constant  Value=2^(31)/180  SampleTime=0.04
  Constant14 : Constant  Value=2^(31)/180  SampleTime=0.04
  Constant2 : Constant  Value=1060  SampleTime=0.04
  Constant7 : Constant  Value=5  SampleTime=0.04
  Constant8 : Constant  SampleTime=0.04
  Constant9 : Constant  SampleTime=0.04
  Data Type Conversion : DataTypeConversion  OutDataTypeStr=boolean  SaturateOnIntegerOverflow=off  RndMeth=Floor
  Data Type Conversion1 : DataTypeConversion  OutDataTypeStr=uint32  SaturateOnIntegerOverflow=off  RndMeth=Floor
  Data Type Conversion{5..8,12..13} (6 alike) : DataTypeConversion  OutDataTypeStr=double  SaturateOnIntegerOverflow=off  RndMeth=Floor
  Data Type Conversion2 : DataTypeConversion  OutDataTypeStr=uint16  SaturateOnIntegerOverflow=off  RndMeth=Floor
  Data Type Conversion33 : DataTypeConversion  OutDataTypeStr=int16  SaturateOnIntegerOverflow=off  RndMeth=Floor
  Data Type Conversion34 : DataTypeConversion  OutDataTypeStr=int16  SaturateOnIntegerOverflow=off  RndMeth=Floor
  Data Type Conversion41 : DataTypeConversion  OutDataTypeStr=boolean  SaturateOnIntegerOverflow=off  RndMeth=Floor
  Data Type Conversion42 : DataTypeConversion  OutDataTypeStr=uint16  SaturateOnIntegerOverflow=off  RndMeth=Floor
  Data Type Conversion43 : DataTypeConversion  OutDataTypeStr=boolean  SaturateOnIntegerOverflow=off  RndMeth=Floor
  Divide3 : Product  Inputs=/*
  Divide4 : Product  Inputs=/*
  Gain19 : Gain  Gain=2^(-20)
  Gain20 : Gain  Gain=2^(-20)
  Gain22 : Gain  Gain=2^(-20)
  Gain4 : Gain  Gain=2^(2)
  Length Conversion{1,15..17,19..20} (6 alike) : aerolibconvert2/Length Conversion  IU=ft  OU=m
  NOT : Logic  Operator=NOT  IconShape=distinctive  AllPortsSameDT=off  OutDataTypeStr=boolean
  GPS_data : Outport  SampleTime=0.04
  wires:
  Length Conversion1/1 -> Bus Creator/5  "Altitude_GPS"
  Bus Selector/7 -> Data Type Conversion12/1  "<VelocityNorth>"
  Bus Selector/2 -> Data Type Conversion1/1  "<GPSTimeOfValidity>"
  Bus Selector/3 -> Data Type Conversion5/1  "<Latitude>"
  Gain4/1 -> Add1/1
  Data Type Conversion33/1 -> Bus Creator/10  "GPSEstHorErr"
  Bus Selector/5 -> Data Type Conversion7/1  "<Altitude>"
  Data Type Conversion8/1 -> Gain22/1
  Data Type Conversion41/1 -> Bus Creator/13  "C_code"
  Bus Selector/11 -> Length Conversion20/1  "<EstimatedVerticalPositionError>"
  Gain20/1 -> Length Conversion16/1
  Bus Selector/10 -> Length Conversion19/1  "<EstimatedHorizontalPositionError>"
  Divide3/1 -> Bus Creator/3  "Latitude_GPS"
  Bus Selector/6 -> Data Type Conversion8/1  "<VelocityEast>"
  Data Type Conversion13/1 -> Gain19/1
  Data Type Conversion6/1 -> Divide4/2
  Data Type Conversion34/1 -> Bus Creator/11  "GPSEstVerticalErr"
  Data Type Conversion42/1 -> Bus Creator/12  "GPS_State"
  Gain22/1 -> Length Conversion15/1
  Length Conversion20/1 -> Data Type Conversion34/1
  Data Type Conversion5/1 -> Divide3/2
  Add1/1 -> Length Conversion1/1
  Data Type Conversion1/1 -> Bus Creator/2  "GPStimeValid"
  Gain19/1 -> Length Conversion17/1
  Constant8/1 -> Data Type Conversion41/1
  Data Type Conversion2/1 -> Bus Creator/9  "FigureofMerit"
  Data Type Conversion7/1 -> Gain4/1
  Bus Selector/8 -> Data Type Conversion13/1  "<VelocityUp>"
  Constant7/1 -> Data Type Conversion42/1
  Bus Selector/4 -> Data Type Conversion6/1  "<Longitude>"
  Bus Selector/9 -> Data Type Conversion2/1  "<GPSStatusFOM>"
  Length Conversion17/1 -> Bus Creator/8  "VelocityUp"
  Length Conversion16/1 -> Bus Creator/7  "VelocityNorth"
  Bus Creator/1 -> GPS_data/1  "GPS"
  Data Type Conversion12/1 -> Gain20/1
  Constant2/1 -> Add1/2
  Length Conversion15/1 -> Bus Creator/6  "VelocityEast"
  Length Conversion19/1 -> Data Type Conversion33/1
  Divide4/1 -> Bus Creator/4  "Longitude_GPS"
  Constant9/1 -> Data Type Conversion43/1
  In_GPS/1 -> Bus Selector/1
  Constant14/1 -> Divide4/1
  Constant12/1 -> Divide3/1
  Data Type Conversion43/1 -> Bus Creator/14  "P_code"
  Data Type Conversion/1 -> NOT/1
  Bus Selector/1 -> Data Type Conversion/1  "<GPSModeWord>"
  NOT/1 -> Bus Creator/1  "GPSDataNotValid"

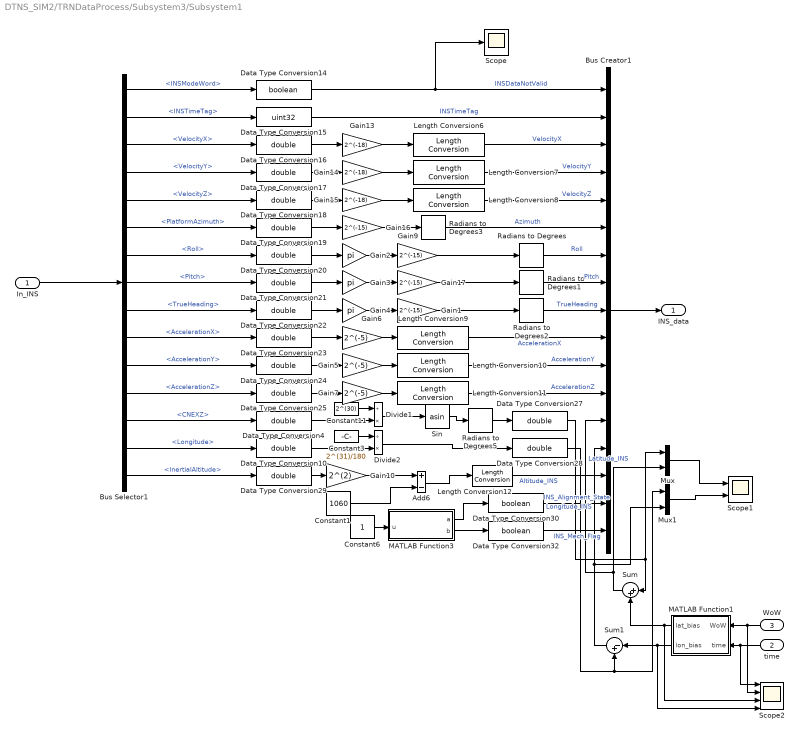
== system DTNS_SIM2/TRNDataProcess/Subsystem3/Subsystem1 ==
  In_INS : Inport  SampleTime=0.04
  time : Inport  Port=2  SampleTime=0.04
  WoW : Inport  Port=3  SampleTime=0.04
  Add6 : Sum  Inputs=+-
  Bus Creator1 : BusCreator  Inputs=17  OutDataTypeStr=Bus: TRN_INS  NonVirtualBus=on
      settings: InheritFromInputs=off
  Bus Selector1 : BusSelector  OutputSignals=INSModeWord,INSTimeTag,VelocityX,VelocityY,VelocityZ,PlatformAzimuth,Roll,Pitch,TrueHeading,AccelerationX,AccelerationY,AccelerationZ,CNEXZ,Longitude,InertialAltitude
  Constant1 : Constant  Value=1060  SampleTime=0.04
  Constant11 : Constant  Value=2^(30)  SampleTime=0.04
  Constant3 : Constant  Value=2^(31)/180  SampleTime=0.04
  Constant6 : Constant  SampleTime=0.04
  Data Type Conversion{4,10,16..25,27..29} (15 alike) : DataTypeConversion  OutDataTypeStr=double  SaturateOnIntegerOverflow=off  RndMeth=Floor
  Data Type Conversion14 : DataTypeConversion  OutDataTypeStr=boolean  SaturateOnIntegerOverflow=off  RndMeth=Floor
  Data Type Conversion15 : DataTypeConversion  OutDataTypeStr=uint32  SaturateOnIntegerOverflow=off  RndMeth=Floor
  Data Type Conversion30 : DataTypeConversion  OutDataTypeStr=boolean  SaturateOnIntegerOverflow=off  RndMeth=Floor
  Data Type Conversion32 : DataTypeConversion  OutDataTypeStr=boolean  SaturateOnIntegerOverflow=off  RndMeth=Floor
  Divide1 : Product  Inputs=/*
  Divide2 : Product  Inputs=/*
  Gain{1,9,16..17} (4 alike) : Gain  Gain=2^(-15)
  Gain10 : Gain  Gain=2^(2)
  Gain13 : Gain  Gain=2^(-18)
  Gain14 : Gain  Gain=2^(-18)
  Gain15 : Gain  Gain=2^(-18)
  Gain2 : Gain  Gain=pi
  Gain3 : Gain  Gain=pi
  Gain4 : Gain  Gain=pi
  Gain5 : Gain  Gain=2^(-5)
  Gain6 : Gain  Gain=2^(-5)
  Gain7 : Gain  Gain=2^(-5)
  Length Conversion{6..12} (7 alike) : aerolibconvert2/Length Conversion  IU=ft  OU=m
  MATLAB Function1 : MATLAB Function  TreatAsAtomicUnit=on  SystemSampleTime=0.04
  MATLAB Function3 : MATLAB Function  TreatAsAtomicUnit=on  SystemSampleTime=0.04
  Mux : Mux  Inputs=2
  Mux1 : Mux  Inputs=2
  Radians to Degrees{,1..3,5} (5 alike) : simulink_extras/Transformations/Radians to Degrees
  Scope : Scope
  Scope1 : Scope  NumInputPorts=2
  Scope2 : Scope  NumInputPorts=4
  Sin : Trigonometry  Operator=asin
  Sum : Sum  Inputs=|++
  Sum1 : Sum  Inputs=|-+
  INS_data : Outport  SampleTime=0.04
  wires:
  Length Conversion6/1 -> Bus Creator1/3  "VelocityX"
  Constant6/1 -> MATLAB Function3/1(u)
  MATLAB Function3/2(b) -> Data Type Conversion32/1
  Data Type Conversion32/1 -> Bus Creator1/17  "INS_Mech_Flag"
  Data Type Conversion22/1 -> Gain4/1
  Length Conversion9/1 -> Bus Creator1/10  "AccelerationX"
  Data Type Conversion29/1 -> Gain10/1
  Radians to Degrees2/1 -> Bus Creator1/9  "TrueHeading"
  Data Type Conversion16/1 -> Gain13/1
  Data Type Conversion18/1 -> Gain15/1
  Data Type Conversion15/1 -> Bus Creator1/2  "INSTimeTag"
  Bus Selector1/14 -> Data Type Conversion10/1  "<Longitude>"
  Radians to Degrees5/1 -> Data Type Conversion27/1
  Data Type Conversion24/1 -> Gain5/1
  Sin/1 -> Radians to Degrees5/1
  Constant1/1 -> Add6/2
  Gain14/1 -> Length Conversion7/1
  Data Type Conversion14/1 -> Scope/1, Bus Creator1/1  "INSDataNotValid"
  Bus Selector1/5 -> Data Type Conversion18/1  "<VelocityZ>"
  Data Type Conversion25/1 -> Gain7/1
  Divide2/1 -> Data Type Conversion28/1
  MATLAB Function3/1(a) -> Data Type Conversion30/1
  Data Type Conversion19/1 -> Gain16/1
  Bus Selector1/10 -> Data Type Conversion23/1  "<AccelerationX>"
  Data Type Conversion20/1 -> Gain2/1
  Bus Selector1/6 -> Data Type Conversion19/1  "<PlatformAzimuth>"
  Data Type Conversion23/1 -> Gain6/1
  Bus Selector1/7 -> Data Type Conversion20/1  "<Roll>"
  Bus Selector1/2 -> Data Type Conversion15/1  "<INSTimeTag>"
  Bus Selector1/4 -> Data Type Conversion17/1  "<VelocityY>"
  Bus Selector1/3 -> Data Type Conversion16/1  "<VelocityX>"
  Add6/1 -> Length Conversion12/1
  Bus Selector1/15 -> Data Type Conversion29/1  "<InertialAltitude>"
  Bus Selector1/12 -> Data Type Conversion25/1  "<AccelerationZ>"
  Bus Selector1/13 -> Data Type Conversion4/1  "<CNEXZ>"
  Data Type Conversion4/1 -> Divide1/2
  Bus Selector1/9 -> Data Type Conversion22/1  "<TrueHeading>"
  Gain15/1 -> Length Conversion8/1
  Bus Selector1/11 -> Data Type Conversion24/1  "<AccelerationY>"
  Length Conversion12/1 -> Bus Creator1/15  "Altitude_INS"
  Gain6/1 -> Length Conversion9/1
  Data Type Conversion21/1 -> Gain3/1
  Length Conversion8/1 -> Bus Creator1/5  "VelocityZ"
  Data Type Conversion17/1 -> Gain14/1
  Radians to Degrees1/1 -> Bus Creator1/8  "Pitch"
  Length Conversion7/1 -> Bus Creator1/4  "VelocityY"
  Constant3/1 -> Divide2/1
  Gain5/1 -> Length Conversion10/1
  Length Conversion10/1 -> Bus Creator1/11  "AccelerationY"
  Gain7/1 -> Length Conversion11/1
  Radians to Degrees/1 -> Bus Creator1/7  "Roll"
  Divide1/1 -> Sin/1
  Bus Selector1/8 -> Data Type Conversion21/1  "<Pitch>"
  Data Type Conversion10/1 -> Divide2/2
  Data Type Conversion30/1 -> Bus Creator1/16  "INS_Alignment_State"
  Gain10/1 -> Add6/1
  Radians to Degrees3/1 -> Bus Creator1/6  "Azimuth"
  Length Conversion11/1 -> Bus Creator1/12  "AccelerationZ"
  Constant11/1 -> Divide1/1
  Gain16/1 -> Radians to Degrees3/1
  Gain13/1 -> Length Conversion6/1
  Bus Creator1/1 -> INS_data/1
  In_INS/1 -> Bus Selector1/1
  Gain3/1 -> Gain17/1
  Gain4/1 -> Gain1/1
  Gain2/1 -> Gain9/1
  Gain9/1 -> Radians to Degrees/1
  Gain17/1 -> Radians to Degrees1/1
  Gain1/1 -> Radians to Degrees2/1
  Bus Selector1/1 -> Data Type Conversion14/1  "<INSModeWord>"
  Sum/1 -> Bus Creator1/13, Mux/2  "Latitude_INS"
  MATLAB Function1/1(lat_bias) -> Scope2/3, Sum/2
  Sum1/1 -> Mux1/2, Bus Creator1/14  "Longitude_INS"
  MATLAB Function1/2(lon_bias) -> Scope2/4, Sum1/1
  Mux/1 -> Scope1/1
  Mux1/1 -> Scope1/2
  Data Type Conversion27/1 -> Sum/1, Mux/1
  Data Type Conversion28/1 -> Sum1/2, Mux1/1
  WoW/1 -> Scope2/2, MATLAB Function1/1(WoW)
  time/1 -> Scope2/1, MATLAB Function1/2(time)

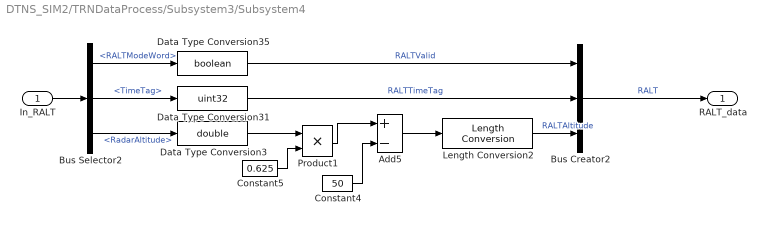
== system DTNS_SIM2/TRNDataProcess/Subsystem3/Subsystem4 ==
  In_RALT : Inport  SampleTime=0.04
  Add5 : Sum  Inputs=+-
  Bus Creator2 : BusCreator  Inputs=3  OutDataTypeStr=Bus: TRN_RALT  NonVirtualBus=on
      settings: InheritFromInputs=off
  Bus Selector2 : BusSelector  OutputSignals=RALTModeWord,TimeTag,RadarAltitude
  Constant4 : Constant  Value=50  SampleTime=0.04
  Constant5 : Constant  Value=0.625  SampleTime=0.04
  Data Type Conversion3 : DataTypeConversion  OutDataTypeStr=double  SaturateOnIntegerOverflow=off  RndMeth=Floor
  Data Type Conversion31 : DataTypeConversion  OutDataTypeStr=uint32  SaturateOnIntegerOverflow=off  RndMeth=Floor
  Data Type Conversion35 : DataTypeConversion  OutDataTypeStr=boolean  SaturateOnIntegerOverflow=off  RndMeth=Floor
  Length Conversion2 : aerolibconvert2/Length Conversion  IU=ft  OU=m
  Product1 : Product
  RALT_data : Outport  SampleTime=0.04
  wires:
  Length Conversion2/1 -> Bus Creator2/3  "RALTAltitude"
  Constant4/1 -> Add5/2
  Bus Creator2/1 -> RALT_data/1  "RALT"
  In_RALT/1 -> Bus Selector2/1
  Data Type Conversion35/1 -> Bus Creator2/1  "RALTValid"
  Add5/1 -> Length Conversion2/1
  Bus Selector2/3 -> Data Type Conversion3/1  "<RadarAltitude>"
  Data Type Conversion3/1 -> Product1/1
  Product1/1 -> Add5/1
  Constant5/1 -> Product1/2
  Data Type Conversion31/1 -> Bus Creator2/2  "RALTTimeTag"
  Bus Selector2/2 -> Data Type Conversion31/1  "<TimeTag>"
  Bus Selector2/1 -> Data Type Conversion35/1  "<RALTModeWord>"

== matlab function DTNS_SIM2/CreateHRInput/ControlHREvent ==
  data: outBus output Bus: HRInput; inBus input Bus: HRInput
function outBus  = ControlHREvent(inBus)
%ControlHREvent
persistent time dt
if isempty(time)
    time = 0.0;
end
if isempty(dt)
    dt = 0.04;
end

ACTIVATED = false;

% Copy
outBus   = inBus;

if ACTIVATED

%     outBus.HRSelected = SET_VALUE(inBus.HRSelected, false, time, 45, 1);

end


time = time + dt;
end


function out = SET_VALUE(in, value, curTime, triggerTime, duration)
out = in;
if (triggerTime <= curTime) && (curTime <= triggerTime+duration)
    out = value;
else
end
end

== matlab function DTNS_SIM2/InitNUpdateMapCache/UpdateCache/UpdateCache ==
  data: result output; lat input; lon input; hDEM output
function [result, hDEM] = UpdateCache(lat, lon)
%UpdateCache

% Persistent variables
persistent latPrev lonPrev
if isempty(latPrev)
    latPrev = 0.0;
end
if isempty(lonPrev)
    lonPrev = 0.0;
end

hDEM = 0.0;

% Initialize output
result = int32(1);

if ( abs(lat - latPrev) > 0.05 ) || ( abs(lon - lonPrev) > 0.05)
    result = coder.ceval('UpdateCache', lat, lon);
    hDEM = coder.ceval('MAPGetTerrainHeight', lat, lon);

    if result == 0
        latPrev = lat;
        lonPrev = lon;
    end
else
    
end

== matlab function DTNS_SIM2/ControlLOSREvent ==
  data: outBus output Bus: LOSRInput; inBus input Bus: LOSRInput
function outBus  = ControlLOSRSimEvent(inBus)
%ControlAGREvent
persistent time dt
if isempty(time)
    time = 0.0;
end
if isempty(dt)
    dt = 0.04;
end

ACTIVATED = false;

% Copy
outBus   = inBus;

if ACTIVATED

    outBus.LOSRSelected = SET_VALUE(inBus.LOSRSelected, false, time, 35, 1);

end


time = time + dt;
end


function out = SET_VALUE(in, value, curTime, triggerTime, duration)
out = in;
if (triggerTime <= curTime) && (curTime <= triggerTime+duration)
    out = value;
else
end
end

== matlab function DTNS_SIM2/InitNUpdateMapCache/InitializeMAP ==
  data: successDTED output; successDVOF output
function [successDTED, successDVOF] = InitializeMAP()
%InitializeMAP

% Persistent variable
persistent firstRun
if isempty(firstRun)
    firstRun = true;
end

% Initialize output
flagDTED = int32(1);
flagDVOF = int32(1);
successDTED = int32(1);
successDVOF = int32(1);

if firstRun
    % Path of DTED data
    pathDTED = 'C:\Users\ASCL\Documents\GitHub\DTNS\MAP\MAP_DB';

    % Length of DETD data path
    strLenDTED = int32(strlength(pathDTED));
    
    % Call [ InitialMap ] : 맵 폴더 위치 설정
    flagDTED = coder.ceval('InitialMap', pathDTED, strLenDTED );
    
    successDTED = flagDTED;

    if (~successDTED)
        firstRun = false;
    end
else
    successDTED = int32(0);
    successDVOF = int32(0);
end

== matlab function DTNS_SIM2/CreateHRInput/BallisticComputer ==
  data: TRNOutput input Bus: TRNOutput; selected output; rangeN output; rangeE output; targetElev input; Valid input
function [selected, rangeN, rangeE] = BallisticComputer(TRNOutput, targetElev, Valid)
%BallisticComputer

% Initialize outputs
selected = true;
rangeN = 0.0;
rangeE = 0.0;

x = 0.0;
z = 0.0;


% Rearrange variables
llh = [TRNOutput.TRNEstOfLatitude; ...
    TRNOutput.TRNEstOfLongitude; ...
    TRNOutput.Altitude_INS - TRNOutput.TRNEstOfINSAltitudeErr];

velXYZ = [TRNOutput.TRN_VelocityX; ...
    TRNOutput.TRN_VelocityY; ...
    TRNOutput.TRN_VelocityZ];

attiDeg = [TRNOutput.TRN_Roll; TRNOutput.TRN_Pitch; TRNOutput.TRN_Yaw];

if Valid
    velNED = body2ned(velXYZ, attiDeg);
    V0 = norm(velNED);
    gamma = atan2d(-velNED(3), sqrt(velNED(1)^2+velNED(2)^2));
    z0 = llh(3);
    x0 = 0;
    T = findTime(double(targetElev), z0, V0, gamma);
    if T >= 0

        heading = atan2d(velNED(2), velNED(1));
        [x, z] = bombKinematics(x0, z0, V0, gamma, T);
        selected = true;
        rangeN = x * cosd(heading);
        rangeE = x * sind(heading);
    else
        selected = false;
        rangeN = 0.0;
        rangeE = 0.0;
    end


else
    selected = true;
    rangeN = 0.0;
    rangeE = 0.0;
end

end

%% Internal functions
function [x, z] = bombKinematics(x0, z0, V0, gamma, t)
    
    g = 9.8;
    x = x0 + V0 * cosd(gamma) .* t;
    z = z0 + V0 * sind(gamma) .* t - 0.5 * g * t.^2;
end

function T = findTime(z, z0, V0, gamma)

g = 9.8;

temp = V0^2*(sind(gamma))^2 - 2*g*(z-z0);

if temp < 0
    T = 0;
else
    T = (V0*sind(gamma) + sqrt(V0^2*(sind(gamma))^2 - 2*g*(z-z0) ) ) / g;
end
end

function [state_eb_n, C_b_n] = body2ned(state_eb_b, eulerDeg)
%body2ned
% Compute the transformation from {Body} frame to local {NED} frame
%
% == Inputs =========
% state_eb_b        - states measured w.r.t. {ECEF} and resolved in {Body}
% eulerDeg          - attitude (euler angles roll-pitch-yaw seq.) [deg]
%
% == Outputs ========
% state_eb_n        - xyz-states resolved in {NED}
% C_b_n             - Transformation matirx from {Body} to {NED} (3x3)
% 

state_eb_n  = zeros(3,1);
C_b_n       = zeros(3,3);

% Body to NED
cRol = cosd(eulerDeg(1));
sRol = sind(eulerDeg(1));
cPit = cosd(eulerDeg(2));
sPit = sind(eulerDeg(2));
cYaw = cosd(eulerDeg(3));
sYaw = sind(eulerDeg(3));
% 
% C_n_b   = [              cPit*cYaw,                cPit*sYaw,     -sPit;...
%           sRol*sPit*cYaw-cRol*sYaw, sRol*sPit*sYaw+cRol*cYaw, sRol*cPit;...
%           cRol*sPit*cYaw+sRol*sYaw, cRol*sPit*sYaw-sRol*cYaw, cRol*cPit];

C_b_n   = [ cPit*cYaw, sRol*sPit*cYaw-cRol*sYaw, cRol*sPit*cYaw+sRol*sYaw;...
            cPit*sYaw, sRol*sPit*sYaw+cRol*cYaw, cRol*sPit*sYaw-sRol*cYaw;...
                -sPit,                sRol*cPit,                cRol*cPit];
% C_b_n   = C_n_b';
      
state_eb_n  = C_b_n * state_eb_b;


end

== matlab function DTNS_SIM2/ControlFlightCmd ==
  data: inBus input Bus: BUS_FLCC_FLIGHT_CMD; outBus output Bus: BUS_FLCC_FLIGHT_CMD; state input
function outBus = ControlFlightCmd(inBus, state)
%ControlFlightCmd
persistent time dt wayPoint
if isempty(time)
    time = 0.0;
end
if isempty(dt)
    dt = 0.01;
end
if isempty(wayPoint)
    wayPoint = 0;
end

ACTIVATED = true;

% -switchGCAS
SWICH_GCAS_NOT_SELECTED = uint8(0);
SWICH_GCAS_SELECTED     = uint8(1);
SWICH_GCAS_AUTO_GCAS    = uint8(2);

% -switchTF
SWICH_TF_NOT_SELECTED   = uint8(0);
SWICH_TF_SELECTED       = uint8(1);
SWICH_TF_AUTO_TF        = uint8(2);

% -switchRoll
SWITCH_ROLL_ATT_HOLD    = uint8(0);
SWITCH_ROLL_STRG_SEL    = uint8(1);
SWITCH_ROLL_HDG_SEL     = uint8(2);

% -switchPitch
SWITCH_PITCH_AP_OFF     = uint8(0);
SWITCH_PITCH_ATT_HOLD   = uint8(1);
SWITCH_PITCH_ALT_HOLD   = uint8(2);

% Copy
outBus = inBus;

if ACTIVATED
    
    % [Roll] Switch
%     outBus.switchRoll = SWITCH_ROLL_ATT_HOLD;
%     outBus.switchRoll = SWITCH_ROLL_STRG_SEL;
    outBus.switchRoll = SWITCH_ROLL_HDG_SEL;

    % [Pitch] Switch
%     outBus.switchPitch = SWITCH_PITCH_AP_OFF;
%     outBus.switchPitch = SWITCH_PITCH_ATT_HOLD;
    outBus.switchPitch = SWITCH_PITCH_ALT_HOLD;

    % [TF] Switch
%     outBus.switchTF = SWICH_TF_NOT_SELECTED;
    outBus.switchTF = SWICH_TF_SELECTED;
%     outBus.switchTF = SWICH_TF_AUTO_TF;

    % [GCAWS] Switch
%     outBus.switchGCAS = SWICH_GCAS_NOT_SELECTED;
%     outBus.switchGCAS = SWICH_GCAS_SELECTED;
    outBus.switchGCAS = SWICH_GCAS_AUTO_GCAS;

    % [WTPG] Sim: Roll
    %     outBus = SET_ATF(outBus, false, time, 0, inf);
    %     outBus = SET_ROLL_ATT(outBus, 30, time, 20, 20);
    %     outBus = SET_ROLL_ATT(outBus, -30, time, 40, 20);
    %     outBus = SET_ROLL_ATT(outBus, 0, time, 60, inf);

    % [DTF & GCAWS] Feasibility Sim
%     outBus.switchTF = SWICH_TF_SELECTED;
%     outBus.switchGCAS = SWICH_GCAS_AUTO_GCAS;
%     outBus.switchRoll = SWITCH_ROLL_ATT_HOLD;
    %     outBus.switchRoll = uint8(0);
    %     outBus.switchPitch = uint8(2);
    %     outBus.refSpeed = SET_VALUE(outBus.refSpeed, 100, time, 0, 40);
    %     outBus.refSpeed = SET_VALUE(outBus.refSpeed, 100, time, 40, 40);

        outBus.nextAlt = 800;
        outBus.refSpeed = 200;
        outBus.switchRoll = SWITCH_ROLL_HDG_SEL;
        outBus.setHeading = 180;

    switch wayPoint
        case 0
            outBus.nextLat = 35.2;
            outBus.nextLon = 128;
        case 1
            outBus.nextLat = 34.8;
            outBus.nextLon = 128.4;
        case 2
            outBus.nextLat = 35.2;
            outBus.nextLon = 128.8;
        case 3
            outBus.nextLat = 37.0;
            outBus.nextLon = 129;
        otherwise
            outBus.nextLat = 37.0;
            outBus.nextLon = 129;
            outBus.nextAlt = 1000;
    end

    if ( abs(state.latitude - outBus.nextLat) < 0.001 ) && ( abs(state.longitude - outBus.nextLon) < 0.001 )
        wayPoint = wayPoint + 1;
    end

    %     outBus.nextAlt = 800.0;

end

% Update Time
time = time + dt;
end

function out = SET_ATF(in, isATF, curTime, triggerTime, duration)
% -switchTF
SWICH_TF_NOT_SELECTED   = uint8(0);
SWICH_TF_SELECTED       = uint8(1);
SWICH_TF_AUTO_TF        = uint8(2);

out = in;
if (triggerTime <= curTime) && (curTime <= triggerTime+duration)
    if isATF
        out.switchTF = SWICH_TF_AUTO_TF;
    else
        out.switchTF = SWICH_TF_SELECTED;
    end

else
end
end

function out = SET_ROLL_ATT(in, rollAngle, curTime, triggerTime, duration)
% -switchRoll
SWITCH_ROLL_ATT_HOLD    = uint8(0);
SWITCH_ROLL_STRG_SEL    = uint8(1);
SWITCH_ROLL_HDG_SEL     = uint8(2);

out = in;
if (triggerTime <= curTime) && (curTime <= triggerTime+duration)
    out.switchRoll = SWITCH_ROLL_ATT_HOLD;
    out.setRoll = rollAngle;
else
end
end

function out = SET_VALUE(in, value, curTime, triggerTime, duration)
out = in;
if (triggerTime <= curTime) && (curTime <= triggerTime+duration)
    out = value;
else
end
end

== matlab function DTNS_SIM2/ControlCREvent ==
  data: outBus output Bus: CRInput; inBus input Bus: CRInput
function outBus  = ControlCREvent(inBus)
%ControlCREvent
persistent time dt
if isempty(time)
    time = 0.0;
end
if isempty(dt)
    dt = 0.04;
end

ACTIVATED = false;

% Copy
outBus   = inBus;

if ACTIVATED

%     outBus.CRSelected = SET_VALUE(inBus.CRSelected, false, time, 55, 1);

end


time = time + dt;
end


function out = SET_VALUE(in, value, curTime, triggerTime, duration)
out = in;
if (triggerTime <= curTime) && (curTime <= triggerTime+duration)
    out = value;
else
end
end

== matlab function DTNS_SIM2/ControlGCAWSInput ==
  data: inBus input Bus: GCAWSInput; GCAWWSInput output Bus: GCAWSInput
function GCAWWSInput = ControlGCAWSInput(inBus)
%ControlGCAWSInput
persistent time dt
if isempty(time)
    time = 0.0;
end
if isempty(dt)
    dt = 0.01;
end
% -------------------------------------------------------------------------
% CONTROL flag
CONTROL_ACTIVATED = true;

% Copy
GCAWWSInput = inBus;

if CONTROL_ACTIVATED
    % Default
    GCAWWSInput.selected        = SET_VALUE(GCAWWSInput.selected,       true, time, 0, inf);
    GCAWWSInput.paramSelected   = SET_VALUE(GCAWWSInput.paramSelected,  true, time, 0, inf);
    GCAWWSInput.reactionTime        = SET_VALUE(GCAWWSInput.reactionTime,       uint16(3), time, 0, inf);
    GCAWWSInput.rollRate            = SET_VALUE(GCAWWSInput.rollRate,           uint16(3), time, 0, inf);
    GCAWWSInput.gOnsetRate          = SET_VALUE(GCAWWSInput.gOnsetRate,         uint16(3), time, 0, inf);
    GCAWWSInput.pullUpG             = SET_VALUE(GCAWWSInput.pullUpG,            uint16(3), time, 0, inf);
    GCAWWSInput.maxFlightPathAngle  = SET_VALUE(GCAWWSInput.maxFlightPathAngle, uint16(3), time, 0, inf);
    GCAWWSInput.gsAvailable         = SET_VALUE(GCAWWSInput.gsAvailable, 5.0, time, 0, inf);
    GCAWWSInput.gsAvaliableValid    = SET_VALUE(GCAWWSInput.gsAvaliableValid, true, time, 0, inf);
    GCAWWSInput.swh                 = SET_VALUE(GCAWWSInput.swh, single(100), time, 0, inf);

    % Control
%     outBus.msd = SET_VALUE(outBus.msd, 500, time, 100, 50);
%     outBus.msd = SET_VALUE(outBus.msd, 500, time, 200, 50);

end

% Update Time
time = time + dt;
end

function out = SET_VALUE(in, value, curTime, triggerTime, duration)
out = in;
if (triggerTime <= curTime) && (curTime <= triggerTime+duration)
    out = value;
else
end
end
